simulink model "questao7_naoseioquetofazendo"  (R2022b)
settings: Solver=VariableStepAuto  StartTime=0.0  StopTime=10.0  RelTol=1e-3
model workspace (MAT data in the model file):
  M = Simulink.Parameter
  M.Value = 540
  M.DataType = 'auto'
  M.Complexity = 'real'
  M.Dimensions = [1 1]
  b = Simulink.Parameter
  b.Value = 1.3
  b.DataType = 'auto'
  b.Complexity = 'real'
  b.Dimensions = [1 1]
  l = Simulink.Parameter
  l.Value = 1.3
  l.DataType = 'auto'
  l.Complexity = 'real'
  l.Dimensions = [1 1]
  m = Simulink.Parameter
  m.Value = 120
  m.DataType = 'auto'
  m.Complexity = 'real'
  m.Dimensions = [1 1]
settings Model: Creator=maria  LastModifiedBy=maria

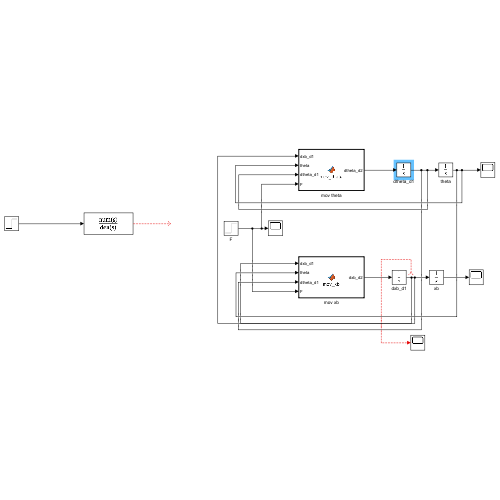
[thumbnail: Simulink's stored preview of the top-level diagram]
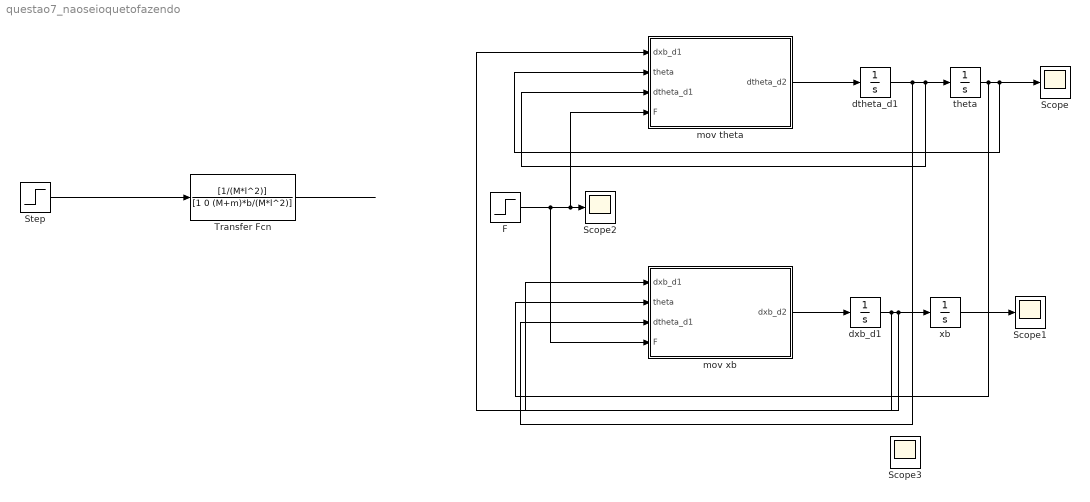
== system questao7_naoseioquetofazendo ==
  F : Step  Time=4  After=540  SampleTime=0
  Scope{,1..3} (4 alike) : Scope
  Step : Step  SampleTime=0
  Transfer Fcn : TransferFcn  Numerator=[1/(M*l^2)]  Denominator=[1 0 (M+m)*b/(M*l^2)]
  dtheta_d1 : Integrator
  dxb_d1 : Integrator
  mov theta : MATLAB Function  TreatAsAtomicUnit=on
  mov xb : MATLAB Function  TreatAsAtomicUnit=on
  theta : Integrator
  xb : Integrator
  wires:
  Transfer Fcn/1 -> ?
  ? -> Scope3/1
  theta/1 -> mov xb/2(theta), mov theta/2(theta), Scope/1
  F/1 -> mov xb/4(F), mov theta/4(F), Scope2/1
  mov theta/1(dtheta_d2) -> dtheta_d1/1
  xb/1 -> Scope1/1
  dxb_d1/1 -> mov xb/1(dxb_d1), mov theta/1(dxb_d1), xb/1
  mov xb/1(dxb_d2) -> dxb_d1/1
  dtheta_d1/1 -> mov xb/3(dtheta_d1), mov theta/3(dtheta_d1), theta/1
  Step/1 -> Transfer Fcn/1

== matlab function questao7_naoseioquetofazendo/mov xb ==
  data: dxb_d1 input; dxb_d2 output; theta input; dtheta_d1 input; F input
function dxb_d2 = mov_xb(dxb_d1, theta, dtheta_d1, F)
    g = 9.81; % m/s^2
    l = 1.30; % m
    m = 120; % kg
    M = 54; % kg
    b = 1.3; % atrito viscoso com o ar
    d = 97.2; % Ns/M
    
    dxb_d2 = (F-d*dxb_d1-m*l*sin(theta)*dtheta_d1^2+m*g*sin(theta)*cos(theta)-(b*dtheta_d1*cos(theta))/l)/((M+m*(sin(theta))^2));

== matlab function questao7_naoseioquetofazendo/mov theta ==
  data: dxb_d1 input; dtheta_d2 output; theta input; dtheta_d1 input; F input
function dtheta_d2 = mov_theta(dxb_d1, theta, dtheta_d1, F)
    g = 9.81; % m/s^2
    l = 1.30; % m
    m = 120; % kg
    M = 54; % kg
    b = 1.3; % atrito viscoso com o ar
    d = 97.2; % Ns/M
    
    dtheta_d2 = ((M+m)*g*l*sin(theta)+l*cos(theta)*(F-d*dxb_d1-m*l*sin(theta)*dtheta_d1^2)-((M+m)*b*dtheta_d1)/m)/(l^2*(M+m*(sin(theta))^2));
